simulink model "Mainframe"  (R2021a)
settings: Solver=FixedStepAuto  StartTime=0.0  StopTime=60  FixedStep=0.001  RelTol=1e-3
values from neighbouring files (symbols this model uses):
  den_lpf_d = den_lpf20    [Mainframe_init.m]    (also in load_autopilot.m)
  Emulated_FCC_IO_Delay = 7    [Mainframe_init.m]
  Enable_Gyros = 0    [Mainframe_init.m]
  Enable_INS = 0    [Mainframe_init.m]
  num_lpf_d = num_lpf20    [Mainframe_init.m]    (also in load_autopilot.m)
undefined symbols (not defined in the file or in its folder): act_dmp, act_omega, Actuator, Aerodynamics, aMode, Autopilot, AUX, c_b_WGS, c_be, c_flat, c_grav, c_h_geop0, c_h_geope, c_pa0, c_pe, c_r0, c_rot, c_rsma, c_Tmp0, d_siB_0, d_siB_max, d_siB_min, dd_siB_max, dd_siB_min, dev, DiscIntNeverNeededParam, e_pa, e_Tmp, fin_maxrate, flag_I_act_switch, flag_I_aero_switch, flag_I_flat, flag_I_gravity_switch, flag_I_rot, hcr, HIL_Data, JMMM_0, JMMM_e, JSPB_e, lat_0, lon_0, Mass_Props, mB_0, mM_0, mM_e, National_Instruments, Newton, pBII_0, PCIe, pMPB, pNPB, propellant_kg, prp_FBPB, prp_mdot, prp_T, pSPB, pwm_output1, qEG_0, qIB_0, qIE_0 ... (+31)
libraries: simulink_extras x38, simulink x31, custom_blocks x11, sldrtlib x10, aerolibcommonsys x4, px4Sensorslib x3, px4lib x3, aerolibnav x1
(part 4 of 17)

== system Mainframe/Flight Simulator On/Flat Earth to LLA/LatLong wrap/Latitude Wrap 90 ==
  Lat : Inport
  Abs1 : Abs
  Bias : Bias  Bias=-90
  Bias1 : Bias  Bias=+90
  Compare To Constant : Subsystem  mask(Compare To Constant){relop=>, const=90, OutDataTypeStr=boolean, ZeroCross=on}
      mask prompts: relop "Simulink:masks:Operator_MP"; const "Simulink:masks:ConstantValue_MP"; OutDataTypeStr "Simulink:masks:OutputDataType_MP"; ZeroCross "Simulink:masks:EnableZerocrossingDetection_MP"
      mask help: Simulink:masks:CompareToConstant_MD
      mask init: same as Mainframe/Non-linear Flight Dynamic Model/Stop-Condition/Compare To Constant
      mask TypeOptions relop: == | ~= | < | <= | >= | >
      mask TypeOptions OutDataTypeStr: Simulink:masks:uint8 | Simulink:masks:boolean
      mask Callback ZeroCross: sl('zeroCrossEnable', gcbh);
      mask Display: disp(str)
  Divide1 : Product  Inputs=**
  Gain : Gain  Gain=-1
  Sign1 : Signum
  Switch : Switch  Criteria=u2 ~= 0
  Wrap Angle 180 : Subsystem
      mask init:
      | aeroicon('aeroblk');
  Lat wrapped : Outport  VectorParamsAs1DForOutWhenUnconnected=off
  Wrap flag : Outport  Port=2  VectorParamsAs1DForOutWhenUnconnected=off
  wires:
  Compare To Constant/1(y) -> Switch/2, Wrap flag/1
  Wrap Angle 180/1(Angle 180) -> Sign1/1, Switch/3, Abs1/1
  Lat/1 -> Wrap Angle 180/1(Angle)
  Abs1/1 -> Compare To Constant/1(u), Bias/1
  Bias/1 -> Gain/1
  Gain/1 -> Bias1/1
  Bias1/1 -> Divide1/2
  Sign1/1 -> Divide1/1
  Divide1/1 -> Switch/1
  Switch/1 -> Lat wrapped/1

== system Mainframe/Flight Simulator On/Flat Earth to LLA/LatLong wrap/Wrap Longitude ==
  Angle : Inport
  Abs : Abs
  Bias : Bias  Bias=180
  Bias1 : Bias  Bias=-180
  Compare To Constant : Subsystem  mask(Compare To Constant){relop=>, const=180, OutDataTypeStr=boolean, ZeroCross=on}
      mask prompts: relop "Simulink:masks:Operator_MP"; const "Simulink:masks:ConstantValue_MP"; OutDataTypeStr "Simulink:masks:OutputDataType_MP"; ZeroCross "Simulink:masks:EnableZerocrossingDetection_MP"
      mask help: Simulink:masks:CompareToConstant_MD
      mask init: same as Mainframe/Non-linear Flight Dynamic Model/Stop-Condition/Compare To Constant
      mask TypeOptions relop: == | ~= | < | <= | >= | >
      mask TypeOptions OutDataTypeStr: Simulink:masks:uint8 | Simulink:masks:boolean
      mask Callback ZeroCross: sl('zeroCrossEnable', gcbh);
      mask Display: disp(str)
  Constant2 : Constant  Value=360
  Math Function1 : Math  Operator=mod  SignedPower=on  SaturateOnIntegerOverflow=on
  Switch : Switch  Criteria=u2 ~= 0  Threshold=180
  Angle 180 : Outport  VectorParamsAs1DForOutWhenUnconnected=off
  wires:
  Compare To Constant/1(y) -> Switch/2
  Angle/1 -> Bias/1, Switch/3, Abs/1
  Abs/1 -> Compare To Constant/1(u)
  Bias/1 -> Math Function1/1
  Constant2/1 -> Math Function1/2
  Math Function1/1 -> Bias1/1
  Bias1/1 -> Switch/1
  Switch/1 -> Angle 180/1

== system Mainframe/Flight Simulator On/Flat Earth to LLA/LatLong wrap1/Latitude Wrap 90 ==
  Lat : Inport
  Abs1 : Abs
  Bias : Bias  Bias=-90
  Bias1 : Bias  Bias=+90
  Compare To Constant : Subsystem  mask(Compare To Constant){relop=>, const=90, OutDataTypeStr=boolean, ZeroCross=on}
      mask prompts: relop "Simulink:masks:Operator_MP"; const "Simulink:masks:ConstantValue_MP"; OutDataTypeStr "Simulink:masks:OutputDataType_MP"; ZeroCross "Simulink:masks:EnableZerocrossingDetection_MP"
      mask help: Simulink:masks:CompareToConstant_MD
      mask init: same as Mainframe/Non-linear Flight Dynamic Model/Stop-Condition/Compare To Constant
      mask TypeOptions relop: == | ~= | < | <= | >= | >
      mask TypeOptions OutDataTypeStr: Simulink:masks:uint8 | Simulink:masks:boolean
      mask Callback ZeroCross: sl('zeroCrossEnable', gcbh);
      mask Display: disp(str)
  Divide1 : Product  Inputs=**
  Gain : Gain  Gain=-1
  Sign1 : Signum
  Switch : Switch  Criteria=u2 ~= 0
  Wrap Angle 180 : Subsystem
      mask init:
      | aeroicon('aeroblk');
  Lat wrapped : Outport  VectorParamsAs1DForOutWhenUnconnected=off
  Wrap flag : Outport  Port=2  VectorParamsAs1DForOutWhenUnconnected=off
  wires:
  Compare To Constant/1(y) -> Switch/2, Wrap flag/1
  Wrap Angle 180/1(Angle 180) -> Sign1/1, Switch/3, Abs1/1
  Lat/1 -> Wrap Angle 180/1(Angle)
  Abs1/1 -> Compare To Constant/1(u), Bias/1
  Bias/1 -> Gain/1
  Gain/1 -> Bias1/1
  Bias1/1 -> Divide1/2
  Sign1/1 -> Divide1/1
  Divide1/1 -> Switch/1
  Switch/1 -> Lat wrapped/1

== system Mainframe/Flight Simulator On/Flat Earth to LLA/LatLong wrap1/Wrap Longitude ==
  Angle : Inport
  Abs : Abs
  Bias : Bias  Bias=180
  Bias1 : Bias  Bias=-180
  Compare To Constant : Subsystem  mask(Compare To Constant){relop=>, const=180, OutDataTypeStr=boolean, ZeroCross=on}
      mask prompts: relop "Simulink:masks:Operator_MP"; const "Simulink:masks:ConstantValue_MP"; OutDataTypeStr "Simulink:masks:OutputDataType_MP"; ZeroCross "Simulink:masks:EnableZerocrossingDetection_MP"
      mask help: Simulink:masks:CompareToConstant_MD
      mask init: same as Mainframe/Non-linear Flight Dynamic Model/Stop-Condition/Compare To Constant
      mask TypeOptions relop: == | ~= | < | <= | >= | >
      mask TypeOptions OutDataTypeStr: Simulink:masks:uint8 | Simulink:masks:boolean
      mask Callback ZeroCross: sl('zeroCrossEnable', gcbh);
      mask Display: disp(str)
  Constant2 : Constant  Value=360
  Math Function1 : Math  Operator=mod  SignedPower=on  SaturateOnIntegerOverflow=on
  Switch : Switch  Criteria=u2 ~= 0  Threshold=180
  Angle 180 : Outport  VectorParamsAs1DForOutWhenUnconnected=off
  wires:
  Compare To Constant/1(y) -> Switch/2
  Angle/1 -> Bias/1, Switch/3, Abs/1
  Abs/1 -> Compare To Constant/1(u)
  Bias/1 -> Math Function1/1
  Constant2/1 -> Math Function1/2
  Math Function1/1 -> Bias1/1
  Bias1/1 -> Switch/1
  Switch/1 -> Angle 180/1

== system Mainframe/Flight Simulator On/Flat Earth to LLA/LongLat_offset/Angle Conversion2 ==
  in : Inport  Unit=deg
  Unit Conversion : UnitConversion
  out : Outport  Unit=rad  VectorParamsAs1DForOutWhenUnconnected=off
  wires:
  Unit Conversion/1 -> out/1
  in/1 -> Unit Conversion/1

== system Mainframe/Flight Simulator On/Flat Earth to LLA/LongLat_offset/Find Radian//Distance ==
  mu : Inport
  Angle Conversion2 : Subsystem
  Constant : Constant
  Constant1 : Constant  Value=R
  Constant2 : Constant
  Constant3 : Constant
  Product1 : Product  Inputs=*/  RndMeth=Zero
  Product2 : Product  RndMeth=Zero
  Product3 : Product  Inputs=**/  RndMeth=Zero
  Product4 : Product  RndMeth=Zero
  Sum1 : Sum  Inputs=|+-
  Trigonometric Function : Trigonometry  Operator=cos
  Trigonometric Function1 : Trigonometry  Operator=atan2
  Trigonometric Function2 : Trigonometry  Operator=atan2
  denom : Subsystem
  e : Subsystem
  e^4 : Subsystem
  sqrt : Sqrt  AlgorithmType=Newton-Raphson  SaturateOnIntegerOverflow=on
  dNorth : Outport  VectorParamsAs1DForOutWhenUnconnected=off
  dEast : Outport  Port=2  VectorParamsAs1DForOutWhenUnconnected=off
  wires:
  Angle Conversion2/1(out) -> Trigonometric Function/1, denom/2(mu)
  Trigonometric Function2/1 -> dEast/1
  Trigonometric Function1/1 -> dNorth/1
  Constant3/1 -> Trigonometric Function2/1
  Constant2/1 -> Trigonometric Function1/1
  Product4/1 -> Trigonometric Function2/2
  mu/1 -> Angle Conversion2/1(in)
  Trigonometric Function/1 -> Product4/2
  Product3/1 -> Trigonometric Function1/2  "Rm"
  Sum1/1 -> Product3/2
  Product1/1 -> Product4/1, Product3/1  "Rn"
  Constant/1 -> Sum1/1
  Product2/1 -> Sum1/2
  Constant1/1 -> Product1/1
  sqrt/1 -> Product1/2
  denom/1(denom) -> sqrt/1, Product3/3
  e^4/1(eps) -> Product2/2, Product2/1, denom/1(eps)
  e/1(e) -> e^4/1(e)

== system Mainframe/Flight Table/Flight Table On/Configure Gimbals/Subsystem ==
  Current Stage : Sum  Inputs=3
  One : Constant  OutDataTypeStr=Inherit: Inherit via back propagation
  Stage : Outport
  wires:
  [stage2complete] -> Current Stage/2
  One/1 -> Current Stage/3
  [stage1complete] -> Current Stage/1
  Current Stage/1 -> Stage/1

== system Mainframe/Flight Table/Flight Table On/Configure Gimbals/Ticks To Degrees ==
  In1 : Inport
  Bus Creator : BusCreator  Inputs=3
  Demux : Demux  Outputs=3
  Shaft2degPitch : Gain  Gain=360/(65536)
  Shaft2degRoll : Gain  Gain=-360/(65536)
  Shaft2degYaw : Gain  Gain=360/(65536)
  Out1 : Outport
  wires:
  Shaft2degYaw/1 -> Bus Creator/1  "yawRaw"
  Shaft2degPitch/1 -> Bus Creator/2  "pitchRaw"
  In1/1 -> Demux/1
  Shaft2degRoll/1 -> Bus Creator/3  "rollRaw"
  Bus Creator/1 -> Out1/1
  Demux/2 -> Shaft2degPitch/1  "pitch"
  Demux/1 -> Shaft2degYaw/1  "yaw"
  Demux/3 -> Shaft2degRoll/1  "roll"

== system Mainframe/Non-linear Flight Dynamic Model/Environment/atm_dynamic/trafo_around_z_axis ==
  vec1 : Inport
  gamma : Inport  Port=2
  1_rot_mat : Subsystem  mask(Rotation um 1, 2 oder 3 Achsen){rot_1=Rotation um z-Achse}
      mask prompts: rot_1 "1. Rotation"
      mask help:
      | Dieser Block liefert die Rotationsmatrix T12 für den Fall zurück, dass sich das Ziel-Koordinatensystem (1) durch Drehungen um 1, 2 oder 3 Achsen gegenüber dem Ausgangskoordinatensystem (2) beschreiben lässt (passive Drehung).
      |
      | Die Anzahl der Rotation sowie die Reihenfolge ist frei einstellbar.
      |
      | Die Rotationswinkel haben die Einheit [rad].
      mask TypeOptions rot_1: Rotation um x-Achse | Rotation um y-Achse | Rotation um z-Achse
  Product : Product  Multiplication=Matrix(*)
  Reshape : Reshape  OutputDimensionality=Column vector (2-D)
  vec2 : Outport  VectorParamsAs1DForOutWhenUnconnected=off
  wires:
  Product/1 -> vec2/1  "vec2"
  gamma/1 -> 1_rot_mat/1(wi1)  "gamma"
  1_rot_mat/1(T12) -> Product/1  "T12"
  vec1/1 -> Reshape/1  "vec1"
  Reshape/1 -> Product/2  "vec1"

== system Mainframe/Non-linear Flight Dynamic Model/Extract States/Assemble_States_Bus1/Rotation Angles to Quaternions ==
  "R1, R2, R3" : Inport  Unit=rad
  1/2 : Gain  Gain=0.5  SaturateOnIntegerOverflow=on  OutDataTypeStr=Inherit: Same as input  ParamDataTypeStr=Inherit: Same as input
  Mux1 : Mux  Inputs=2
  Mux2 : Mux
  q0 : Fcn  Expr=u(4)*u(5)*u(6) + u(1)*u(2)*u(3)
  q1 : Fcn  Expr=u(4)*u(5)*u(3) - u(1)*u(2)*u(6)
  q2 : Fcn  Expr=u(4)*u(2)*u(6) + u(1)*u(5)*u(3)
  q3 : Fcn  Expr=u(1)*u(5)*u(6) - u(4)*u(2)*u(3)
  sincos : Trigonometry  Operator=sincos
  Quat : Outport  Unit=1  InitialOutput=0  VectorParamsAs1DForOutWhenUnconnected=off
  wires:
  q0/1 -> Mux2/1
  Mux2/1 -> Quat/1
  q3/1 -> Mux2/4
  q2/1 -> Mux2/3
  q1/1 -> Mux2/2
  Mux1/1 -> q3/1, q2/1, q1/1, q0/1
  sincos/2 -> Mux1/2
  sincos/1 -> Mux1/1
  1/2/1 -> sincos/1
  "R1, R2, R3"/1 -> 1/2/1

== system Mainframe/Non-linear Flight Dynamic Model/Extract States/Assemble_States_Bus1/Three-axis Inertial Measurement Unit3 ==
  A_b : Inport  Unit=m/s^2
  w : Inport  Port=2  Unit=rad/s
  w_dot : Inport  Port=3  Unit=rad/s^2
  CG : Inport  Port=4  Unit=m
  g : Inport  Port=5  Unit=m/s^2
  Acceleration Conversion : Subsystem
  Disallow CGS : UnitConfiguration  UnitSystemsStr=English,SI,SI (extended)  AllowAllUnitSystems=off
  Three-axis Accelerometer : Subsystem  mask(Three-axis Accelerometer){units=Metric (MKS), acc=imu, gtype=on, dtype_a=on, w_a=w_a, z_a=z_a, a_sf_cc=a_sf_cc, a_bias=a_bias, a_Ts=i_Ts, a_rand=on, a_seeds=i_seeds(1:3), a_pow=i_pow(1:3), a_sat=a_sat}
      mask prompts: units "aeroblks:aeroblknav:blockThreeaxisAccelerometerParamUnits"; acc "aeroblks:aeroblknav:blockThreeaxisAccelerometerParamAccelerometerlocation"; gtype "aeroblks:aeroblknav:blockThreeaxisAccelerometerParamSubtractgravity"; dtype_a "aeroblks:aeroblknav:blockThreeaxisAccelerometerParamSecondorderdynamics"; w_a "aeroblks:aeroblknav:blockThreeaxisAccelerometerParamNaturalfrequencyradsec"; z_a "aeroblks:aeroblknav:blockThreeaxisAccelerometerParamDampingratio"; a_sf_cc "aeroblks:aeroblknav:blockThreeaxisAccelerometerParamScalefactorsandcrosscoupling"; a_bias "aeroblks:aeroblknav:blockThreeaxisAccelerometerParamMeasurementbias"; a_Ts "aeroblks:aeroblknav:blockThreeaxisAccelerometerParamUpdateratesec"; a_rand "aeroblks:aeroblknav:blockThreeaxisAccelerometerParamNoiseon"; a_seeds "aeroblks:aeroblknav:blockThreeaxisAccelerometerParamNoiseseeds"; a_pow "aeroblks:aeroblknav:blockThreeaxisAccelerometerParamNoisepower"; a_sat "aeroblks:aeroblknav:blockThreeaxisAccelerometerParamLowerandupperoutputlimits"
      mask help: aeroblks:aeroblknav:blockThreeaxisAccelerometerDesc
      mask init:
      | par = a_Ts;
      | block = gcb;
      | ports=aeroicon('aeroblkaccel','icon',par);
      | a_satl = a_sat(1:3);
      | a_sath = a_sat(4:6);
      mask Help: eval('asbhelp');
      mask TypeOptions units: aeroblks:aeroblknav:blockThreeaxisAccelerometerParamComboMetricMKS | aeroblks:aeroblknav:blockThreeaxisAccelerometerParamComboEnglish
      mask Callback gtype: aeroicon('aeroblkaccel')
      mask Callback dtype_a: aeroicon('aeroblkaccel')
      mask Callback a_rand: aeroicon('aeroblkaccel')
      mask DialogControl ParameterTabVar0 Prompt: Main
      mask DialogControl units Prompt: Units:
      mask DialogControl acc Prompt: Accelerometer location:
      mask DialogControl gtype Prompt: Subtract gravity:
      mask DialogControl dtype_a Prompt: Second-order dynamics
      mask DialogControl w_a Prompt: Natural frequency (rad/sec):
      mask DialogControl z_a Prompt: Damping ratio:
      mask DialogControl a_sf_cc Prompt: Scale factors and cross-coupling:
      mask DialogControl a_bias Prompt: Measurement bias:
      mask DialogControl a_Ts Prompt: Update rate (sec):
      mask DialogControl ParameterTabVar01 Prompt: Noise
      mask DialogControl a_rand Prompt: Noise on
      mask DialogControl a_seeds Prompt: Noise seeds:
      mask DialogControl a_pow Prompt: Noise power:
      mask DialogControl a_sat Prompt: Lower and upper output limits:
      mask Display:
      | port_label(ports(1).type,ports(1).port,ports(1).txt,'texmode','on');
      | port_label(ports(2).type,ports(2).port,ports(2).txt,'texmode','on');
      | port_label(ports(3).type,ports(3).port,ports(3).txt,'texmode','on');
      | port_label(ports(4).type,ports(4).port,ports(4).txt,'texmode','on');
      | port_label(ports(5).type,ports(5).port,ports(5).txt,'texmode','on');
      | port_label(ports(6).type,ports(6).port,ports(6).txt,'texmode','on');
  Three-axis Gyroscope : Subsystem  mask(Three-axis Gyroscope){dtype_g=on, w_g=w_g, z_g=z_g, g_sf_cc=g_sf_cc, g_bias=g_bias, g_sen=g_sens, g_Ts=i_Ts, g_rand=on, g_seeds=i_seeds(4:6), g_pow=i_pow(4:6), g_sat=g_sat}
      mask prompts: dtype_g "aeroblks:aeroblknav:blockThreeaxisGyroscopeParamSecondorderdynamics"; w_g "aeroblks:aeroblknav:blockThreeaxisGyroscopeParamNaturalfrequencyradsec"; z_g "aeroblks:aeroblknav:blockThreeaxisGyroscopeParamDampingratio"; g_sf_cc "aeroblks:aeroblknav:blockThreeaxisGyroscopeParamScalefactorsandcrosscoupling"; g_bias "aeroblks:aeroblknav:blockThreeaxisGyroscopeParamMeasurementbias"; g_sen "aeroblks:aeroblknav:blockThreeaxisGyroscopeParamGsensitivebias"; g_Ts "aeroblks:aeroblknav:blockThreeaxisGyroscopeParamUpdateratesec"; g_rand "aeroblks:aeroblknav:blockThreeaxisGyroscopeParamNoiseon"; g_seeds "aeroblks:aeroblknav:blockThreeaxisGyroscopeParamNoiseseeds"; g_pow "aeroblks:aeroblknav:blockThreeaxisGyroscopeParamNoisepower"; g_sat "aeroblks:aeroblknav:blockThreeaxisGyroscopeParamLowerandupperoutputlimits"
      mask help: aeroblks:aeroblknav:blockThreeaxisGyroscopeDesc
      mask init:
      | par = g_Ts;
      | block = gcb;
      | g_satl = g_sat(1:3);
      | g_sath = g_sat(4:6);
      | ports=aeroicon('aeroblkgyro','icon',par);
      mask Help: eval('asbhelp');
      mask Callback dtype_g: aeroicon('aeroblkgyro');
      mask Callback g_rand: aeroicon('aeroblkgyro');
      mask DialogControl ParameterTabVar0 Prompt: Main
      mask DialogControl dtype_g Prompt: Second-order dynamics
      mask DialogControl w_g Prompt: Natural frequency (rad/sec):
      mask DialogControl z_g Prompt: Damping ratio:
      mask DialogControl g_sf_cc Prompt: Scale factors and cross-coupling:
      mask DialogControl g_bias Prompt: Measurement bias:
      mask DialogControl g_sen Prompt: G-sensitive bias:
      mask DialogControl g_Ts Prompt: Update rate (sec):
      mask DialogControl ParameterTabVar01 Prompt: Noise
      mask DialogControl g_rand Prompt: Noise on
      mask DialogControl g_seeds Prompt: Noise seeds:
      mask DialogControl g_pow Prompt: Noise power:
      mask DialogControl g_sat Prompt: Lower and upper output limits:
      mask Display:
      | port_label(ports(1).type,ports(1).port,ports(1).txt,'texmode','on');
      | port_label(ports(2).type,ports(2).port,ports(2).txt,'texmode','on');
      | port_label(ports(3).type,ports(3).port,ports(3).txt,'texmode','on');
  A_meas : Outport  Unit=m/s^2  VectorParamsAs1DForOutWhenUnconnected=off
  w_meas : Outport  Port=2  Unit=rad/s  VectorParamsAs1DForOutWhenUnconnected=off
  wires:
  Three-axis Accelerometer/1(Ameas) -> A_meas/1
  Three-axis Gyroscope/1((p q r)_meas) -> w_meas/1
  A_b/1 -> Acceleration Conversion/1(acceleration), Three-axis Accelerometer/1(Ab)
  w/1 -> Three-axis Accelerometer/2(p q r), Three-axis Gyroscope/1(p q r)
  CG/1 -> Three-axis Accelerometer/4(CG)
  w_dot/1 -> Three-axis Accelerometer/3(pdot qdot rdot)
  Acceleration Conversion/1(inherit) -> Three-axis Gyroscope/2(G's)
  g/1 -> Three-axis Accelerometer/5(g)

== system Mainframe/Non-linear Flight Dynamic Model/GRM_Airframe/aerodynamics/aerodynamic_via_lookup ==
  pBPB : Inport
  qdynB : Inport  Port=2
  MaB : Inport  Port=3
  alB : Inport  Port=4
  beB : Inport  Port=5
  hBE : Inport  Port=6
  wBIB_star : Inport  Port=7
  afinB : Inport  Port=8
  flag_I_prp : Inport  Port=9
  Bus Creator : BusCreator  Inputs=2
  Demux1 : Demux  Outputs=3
  Demux3 : Demux  Outputs=3
  Gain{,1..4} (5 alike) : Gain  Gain=180/pi
      settings: AttributesFormatString=%<Gain>
  Saturation1 : Saturate  UpperLimit=Aerodynamics.ulim_alpha_deg  LowerLimit=Aerodynamics.llim_alpha_deg
      settings: AttributesFormatString=|
      | %<UpperLimit>
      | %<LowerLimit>
  Saturation4 : Saturate  UpperLimit=Aerodynamics.ulim_beta_deg  LowerLimit=Aerodynamics.llim_beta_deg
      settings: AttributesFormatString=|
      | %<UpperLimit>
      | %<LowerLimit>
  Terminator : Terminator
  Terminator1 : Terminator
  calc_aero_coefficients : Subsystem
  calc_aero_for_mom : Subsystem
  aero_bus : Outport  VectorParamsAs1DForOutWhenUnconnected=off
  wires:
  MaB/1 -> Terminator1/1
  calc_aero_for_mom/1(FBAB) -> Bus Creator/1
  Bus Creator/1 -> aero_bus/1  "aero_bus"
  pBPB/1 -> calc_aero_for_mom/2(pBPB)
  flag_I_prp/1 -> Terminator/1
  hBE/1 -> calc_aero_for_mom/1(hBE)
  calc_aero_for_mom/2(MBAB) -> Bus Creator/2
  qdynB/1 -> calc_aero_for_mom/3(qdynB)
  alB/1 -> Gain3/1
  beB/1 -> Gain4/1
  wBIB_star/1 -> Demux1/1
  Demux1/1 -> calc_aero_coefficients/4(pBIB_star_rps)  "pBIB_star_rps"
  Demux1/2 -> calc_aero_coefficients/5(qBIB_star_rps)  "qBIB_star_rps"
  Demux1/3 -> calc_aero_coefficients/6(rBIB_star_rps)  "rBIB_star_rps"
  afinB/1 -> Demux3/1
  Demux3/2 -> Gain1/1  "etB"
  Demux3/1 -> Gain/1  "xiB"
  Demux3/3 -> Gain2/1  "zeB"
  Gain/1 -> calc_aero_coefficients/1(dela_deg)
  Gain1/1 -> calc_aero_coefficients/2(dele_deg)
  Gain2/1 -> calc_aero_coefficients/3(delr_deg)
  calc_aero_coefficients/1(Cx) -> calc_aero_for_mom/4(Cx)
  calc_aero_coefficients/2(Cy) -> calc_aero_for_mom/5(Cy)
  calc_aero_coefficients/3(Cz) -> calc_aero_for_mom/6(Cz)
  calc_aero_coefficients/4(Cl) -> calc_aero_for_mom/7(Cl)
  calc_aero_coefficients/5(Cm) -> calc_aero_for_mom/8(Cm)
  calc_aero_coefficients/6(Cn) -> calc_aero_for_mom/9(Cn)
  Saturation1/1 -> calc_aero_coefficients/7(alB_deg)
  Saturation4/1 -> calc_aero_coefficients/8(beB_deg)
  Gain3/1 -> Saturation1/1
  Gain4/1 -> Saturation4/1

== system Mainframe/Non-linear Flight Dynamic Model/GRM_Airframe/aerodynamics/logic_base_drag ==
  env_glbl : Inport
  Bus Selector1 : BusSelector  OutputSignals=T_sim_glbl,T_sim_lnch
  Constant : Constant  Value=prp_T(end)
  MATLAB Function : MATLAB Function  TreatAsAtomicUnit=on
  Subtract : Sum  Inputs=+-
  flag_base_drag : Outport  VectorParamsAs1DForOutWhenUnconnected=off
  wires:
  Subtract/1 -> MATLAB Function/1(u)
  Constant/1 -> MATLAB Function/2(t_prp2)
  MATLAB Function/1(flag_base_drag) -> flag_base_drag/1  "flag_base_drag"
  Bus Selector1/1 -> Subtract/1  "<T_sim_glbl>"
  Bus Selector1/2 -> Subtract/2  "<T_sim_lnch>"
  env_glbl/1 -> Bus Selector1/1

== system Mainframe/Non-linear Flight Dynamic Model/GRM_Airframe/environment/WGS84_Gravitation ==
  lon : Inport  PortDimensions=1
  lat : Inport  Port=2  PortDimensions=1
  h : Inport  Port=3  PortDimensions=1
  Assertion : Assertion  AssertionFailFcn="error('WGS84 Gravitationsmodell: Die Werte des Eingangs \"h\" muessen groesser als 0 sein')"
  Assertion1 : Assertion  AssertionFailFcn="error('WGS84 Gravitationsmodell: Die Werte des Eingangs \"Long\" muessen zwischen -180 und +180 liegen')"
  Assertion2 : Assertion  AssertionFailFcn="error('WGS84 Gravitationsmodell: Die Werte des Eingangs \"Lat\" muessen zwischen -90 und +90 liegen')"
  Compare To Constant : simulink/Logic and Bit Operations/Compare To Constant  relop=>=  const=0  OutDataTypeStr=boolean
      settings: SourceProductName=ISim Simulink Block Set
  Interval Test : simulink/Logic and Bit Operations/Interval Test  IntervalClosedRight=on  uplimit=pi  IntervalClosedLeft=on  lowlimit=-pi  OutDataTypeStr=boolean
      settings: SourceProductName=ISim Simulink Block Set
  Interval Test1 : simulink/Logic and Bit Operations/Interval Test  IntervalClosedRight=on  uplimit=pi/2  IntervalClosedLeft=on  lowlimit=-pi/2  OutDataTypeStr=boolean
      settings: SourceProductName=ISim Simulink Block Set
  WGS84_2_ECEF : Subsystem
  WGS84_Gravity_Implementation : MATLAB Function  TreatAsAtomicUnit=on
  gE : Outport  PortDimensions=3  VectorParamsAs1DForOutWhenUnconnected=off
  wires:
  Interval Test1/1 -> Assertion2/1
  Interval Test/1 -> Assertion1/1
  Compare To Constant/1 -> Assertion/1
  WGS84_2_ECEF/1(pE) -> WGS84_Gravity_Implementation/1(pE)  "pE"
  lat/1 -> WGS84_Gravity_Implementation/2(lat_rad), Interval Test1/1, WGS84_2_ECEF/3(lat)  "lat"
  lon/1 -> WGS84_Gravity_Implementation/3(long_rad), Interval Test/1, WGS84_2_ECEF/2(lon)  "lon"
  h/1 -> WGS84_2_ECEF/1(h), Compare To Constant/1  "h"
  WGS84_Gravity_Implementation/1(gamma_R) -> gE/1  "gE"

== system Mainframe/Non-linear Flight Dynamic Model/GRM_Airframe/environment/atmosphere_static_ISO_2533 ==
  hBE : Inport
  env_glbl : Inport  Port=2
  Bus Creator1 : BusCreator  Inputs=6
  Bus Selector1 : BusSelector  OutputSignals=e_Tmp,e_pa
  Saturation : Saturate  UpperLimit=c_h_geope  LowerLimit=c_h_geop0
      settings: AttributesFormatString=|
      | %<UpperLimit>
      | %<LowerLimit>
  density : Subsystem
  geopot_height : Subsystem  mask{mean_earth_radius=c_r0}
      mask prompts: mean_earth_radius "Mean Earth Radius WGS 84 [m]"
      mask TypeOptions mean_earth_radius: mean_earth_radius/Value
  speed_of_sound : Subsystem
  tmp_and_pressure_ISO_2533 : Subsystem
  atm_stat : Outport  VectorParamsAs1DForOutWhenUnconnected=off
  wires:
  speed_of_sound/1(sos) -> Bus Creator1/3
  env_glbl/1 -> Bus Selector1/1
  Bus Selector1/2 -> tmp_and_pressure_ISO_2533/3(e_pa)  "<e_pa>"
  geopot_height/1(h_geop) -> Saturation/1
  Bus Selector1/1 -> tmp_and_pressure_ISO_2533/2(e_Tmp)  "<e_Tmp>"
  Bus Creator1/1 -> atm_stat/1  "atm_stat_bus"
  tmp_and_pressure_ISO_2533/1(Tmp) -> speed_of_sound/1(Tmp), Bus Creator1/4, density/1(Tmp)
  tmp_and_pressure_ISO_2533/2(pa) -> Bus Creator1/6, density/2(pa)
  density/1(rho) -> Bus Creator1/5
  hBE/1 -> Bus Creator1/1, geopot_height/1(hBE)
  Saturation/1 -> Bus Creator1/2, tmp_and_pressure_ISO_2533/1(h_geop)  "h_geop"

== system Mainframe/Non-linear Flight Dynamic Model/GRM_Airframe/environment/convert_to_local_frame ==
  gE : Inport
  Constant1 : Constant  Value=0
  Dot Product : DotProduct  InputSameDT=on  OutDataTypeStr=Inherit: Inherit via internal rule
  Sqrt : Sqrt  SaturateOnIntegerOverflow=on
  Vector Concatenate : Concatenate  NumInputs=3  Mode=Multidimensional array
  gBG : Outport  VectorParamsAs1DForOutWhenUnconnected=off
  wires:
  gE/1 -> Dot Product/1, Dot Product/2
  Constant1/1 -> Vector Concatenate/2, Vector Concatenate/1
  Sqrt/1 -> Vector Concatenate/3
  Vector Concatenate/1 -> gBG/1  "gBG"
  Dot Product/1 -> Sqrt/1

== system Mainframe/Non-linear Flight Dynamic Model/GRM_Airframe/fin_actuators/Rudder ==
  siB_c : Inport
  tRRR : Inport  Port=2
  Add : Sum  Inputs=+-
  Add1 : Sum  Inputs=+-
  Add2 : Sum  Inputs=+++
  Constant1 : Constant  Value=Actuator.fin1_bias
      settings: AttributesFormatString=%<Value>
  Gain : Gain  Gain=omega^2
  Gain2 : Gain  Gain=2*dmp*omega  Multiplication=Matrix(K*u)
  Gain3 : Gain  Gain=unc_bl
  Gain4 : Gain  Gain=Actuator.fin1_scale
      settings: AttributesFormatString=%<Gain>
  Integrator : Integrator  ExternalReset=either  InitialCondition=d_siB_0
  Integrator1 : Integrator  InitialCondition=siB_0  LimitOutput=on  UpperSaturationLimit=siB_max  LowerSaturationLimit=siB_min  ShowSaturationPort=on
  Limiting_Acceleration : MATLAB Function  TreatAsAtomicUnit=on
  Limiting_Rate : MATLAB Function  TreatAsAtomicUnit=on
  Saturation : Saturate  UpperLimit=siB_max  LowerLimit=siB_min
  Saturation1 : Saturate  UpperLimit=siB_max  LowerLimit=siB_min
  Sign : Signum
  siB : Outport  VectorParamsAs1DForOutWhenUnconnected=off
  d_siB : Outport  Port=2  VectorParamsAs1DForOutWhenUnconnected=off
  dd_siB : Outport  Port=3  VectorParamsAs1DForOutWhenUnconnected=off
  wires:
  Saturation1/1 -> siB/1, [siB]  "siB"
  Integrator1/2 -> Integrator/2  "sat"
  Gain4/1 -> Add2/2
  Gain3/1 -> Add2/3
  Sign/1 -> Gain3/1
  tRRR/1 -> Sign/1  "tRRR"
  Integrator1/1 -> Gain4/1, Add/2  "siB"
  Add1/1 -> Limiting_Acceleration/3(dd_siB)  "dd_siB"
  Gain2/1 -> Add1/2
  Gain/1 -> Add1/1
  Add/1 -> Gain/1
  Limiting_Acceleration/1(dd_siB_l) -> Integrator/1, dd_siB/1  "dd_siB_l"
  Limiting_Rate/1(d_siB_l) -> d_siB/1, [d_siB], Integrator1/1  "d_siB_l"
  Integrator/1 -> Limiting_Rate/2(d_siB), Gain2/1  "d_siB"
  Saturation/1 -> Add/1
  Add2/1 -> Saturation1/1
  Constant1/1 -> Add2/1
  siB_c/1 -> Saturation/1  "siB_c"
  [d_siB] -> Limiting_Acceleration/2(d_siB)
  [siB] -> Limiting_Acceleration/1(siB)
  [siB] -> Limiting_Rate/1(siB)

== system Mainframe/Non-linear Flight Dynamic Model/GRM_Airframe/fin_actuators/Rudder1 ==
  siB_c : Inport
  tRRR : Inport  Port=2
  Add : Sum  Inputs=+-
  Add1 : Sum  Inputs=+-
  Add3 : Sum  Inputs=+++
  Constant1 : Constant  Value=Actuator.fin2_bias
      settings: AttributesFormatString=%<Value>
  Gain : Gain  Gain=omega^2
  Gain2 : Gain  Gain=2*dmp*omega  Multiplication=Matrix(K*u)
  Gain3 : Gain  Gain=unc_bl
  Gain4 : Gain  Gain=Actuator.fin2_scale
      settings: AttributesFormatString=%<Gain>
  Integrator : Integrator  ExternalReset=either  InitialCondition=d_siB_0
  Integrator1 : Integrator  InitialCondition=siB_0  LimitOutput=on  UpperSaturationLimit=siB_max  LowerSaturationLimit=siB_min  ShowSaturationPort=on
  Limiting_Acceleration : MATLAB Function  TreatAsAtomicUnit=on
  Limiting_Rate : MATLAB Function  TreatAsAtomicUnit=on
  Saturation : Saturate  UpperLimit=siB_max  LowerLimit=siB_min
  Saturation1 : Saturate  UpperLimit=siB_max  LowerLimit=siB_min
  Sign : Signum
  siB : Outport  VectorParamsAs1DForOutWhenUnconnected=off
  d_siB : Outport  Port=2  VectorParamsAs1DForOutWhenUnconnected=off
  dd_siB : Outport  Port=3  VectorParamsAs1DForOutWhenUnconnected=off
  wires:
  Saturation1/1 -> siB/1, [siB]  "siB"
  Integrator1/2 -> Integrator/2  "sat"
  Gain3/1 -> Add3/3
  Sign/1 -> Gain3/1
  tRRR/1 -> Sign/1  "tRRR"
  Integrator1/1 -> Add/2, Gain4/1  "siB"
  Add1/1 -> Limiting_Acceleration/3(dd_siB)  "dd_siB"
  Gain2/1 -> Add1/2
  Gain/1 -> Add1/1
  Add/1 -> Gain/1
  Limiting_Acceleration/1(dd_siB_l) -> Integrator/1, dd_siB/1  "dd_siB_l"
  Limiting_Rate/1(d_siB_l) -> d_siB/1, [d_siB], Integrator1/1  "d_siB_l"
  Integrator/1 -> Limiting_Rate/2(d_siB), Gain2/1  "d_siB"
  Saturation/1 -> Add/1
  Add3/1 -> Saturation1/1
  siB_c/1 -> Saturation/1  "siB_c"
  [d_siB] -> Limiting_Acceleration/2(d_siB)
  [siB] -> Limiting_Acceleration/1(siB)
  [siB] -> Limiting_Rate/1(siB)
  Constant1/1 -> Add3/1
  Gain4/1 -> Add3/2

== system Mainframe/Non-linear Flight Dynamic Model/GRM_Airframe/fin_actuators/Rudder2 ==
  siB_c : Inport
  tRRR : Inport  Port=2
  Add : Sum  Inputs=+-
  Add1 : Sum  Inputs=+-
  Add3 : Sum  Inputs=+++
  Constant1 : Constant  Value=Actuator.fin3_bias
      settings: AttributesFormatString=%<Value>
  Gain : Gain  Gain=omega^2
  Gain2 : Gain  Gain=2*dmp*omega  Multiplication=Matrix(K*u)
  Gain3 : Gain  Gain=unc_bl
  Gain4 : Gain  Gain=Actuator.fin3_scale
      settings: AttributesFormatString=%<Gain>
  Integrator : Integrator  ExternalReset=either  InitialCondition=d_siB_0
  Integrator1 : Integrator  InitialCondition=siB_0  LimitOutput=on  UpperSaturationLimit=siB_max  LowerSaturationLimit=siB_min  ShowSaturationPort=on
  Limiting_Acceleration : MATLAB Function  TreatAsAtomicUnit=on
  Limiting_Rate : MATLAB Function  TreatAsAtomicUnit=on
  Saturation : Saturate  UpperLimit=siB_max  LowerLimit=siB_min
  Saturation1 : Saturate  UpperLimit=siB_max  LowerLimit=siB_min
  Sign : Signum
  siB : Outport  VectorParamsAs1DForOutWhenUnconnected=off
  d_siB : Outport  Port=2  VectorParamsAs1DForOutWhenUnconnected=off
  dd_siB : Outport  Port=3  VectorParamsAs1DForOutWhenUnconnected=off
  wires:
  Saturation1/1 -> siB/1, [siB]  "siB"
  Integrator1/2 -> Integrator/2  "sat"
  Gain3/1 -> Add3/3
  Sign/1 -> Gain3/1
  tRRR/1 -> Sign/1  "tRRR"
  Integrator1/1 -> Gain4/1, Add/2  "siB"
  Add1/1 -> Limiting_Acceleration/3(dd_siB)  "dd_siB"
  Gain2/1 -> Add1/2
  Gain/1 -> Add1/1
  Add/1 -> Gain/1
  Limiting_Acceleration/1(dd_siB_l) -> Integrator/1, dd_siB/1  "dd_siB_l"
  Limiting_Rate/1(d_siB_l) -> d_siB/1, [d_siB], Integrator1/1  "d_siB_l"
  Integrator/1 -> Limiting_Rate/2(d_siB), Gain2/1  "d_siB"
  Saturation/1 -> Add/1
  Add3/1 -> Saturation1/1
  siB_c/1 -> Saturation/1  "siB_c"
  [d_siB] -> Limiting_Acceleration/2(d_siB)
  [siB] -> Limiting_Acceleration/1(siB)
  [siB] -> Limiting_Rate/1(siB)
  Constant1/1 -> Add3/1
  Gain4/1 -> Add3/2

== system Mainframe/Non-linear Flight Dynamic Model/GRM_Airframe/fin_actuators/Rudder3 ==
  siB_c : Inport
  tRRR : Inport  Port=2
  Add : Sum  Inputs=+-
  Add1 : Sum  Inputs=+-
  Add3 : Sum  Inputs=+++
  Constant1 : Constant  Value=Actuator.fin4_bias
      settings: AttributesFormatString=%<Value>
  Gain : Gain  Gain=omega^2
  Gain2 : Gain  Gain=2*dmp*omega  Multiplication=Matrix(K*u)
  Gain3 : Gain  Gain=unc_bl
  Gain4 : Gain  Gain=Actuator.fin4_scale
      settings: AttributesFormatString=%<Gain>
  Integrator : Integrator  ExternalReset=either  InitialCondition=d_siB_0
  Integrator1 : Integrator  InitialCondition=siB_0  LimitOutput=on  UpperSaturationLimit=siB_max  LowerSaturationLimit=siB_min  ShowSaturationPort=on
  Limiting_Acceleration : MATLAB Function  TreatAsAtomicUnit=on
  Limiting_Rate : MATLAB Function  TreatAsAtomicUnit=on
  Saturation : Saturate  UpperLimit=siB_max  LowerLimit=siB_min
  Saturation1 : Saturate  UpperLimit=siB_max  LowerLimit=siB_min
  Sign : Signum
  siB : Outport  VectorParamsAs1DForOutWhenUnconnected=off
  d_siB : Outport  Port=2  VectorParamsAs1DForOutWhenUnconnected=off
  dd_siB : Outport  Port=3  VectorParamsAs1DForOutWhenUnconnected=off
  wires:
  Saturation1/1 -> siB/1, [siB]  "siB"
  Integrator1/2 -> Integrator/2  "sat"
  Gain3/1 -> Add3/3
  Sign/1 -> Gain3/1
  tRRR/1 -> Sign/1  "tRRR"
  Integrator1/1 -> Gain4/1, Add/2  "siB"
  Add1/1 -> Limiting_Acceleration/3(dd_siB)  "dd_siB"
  Gain2/1 -> Add1/2
  Gain/1 -> Add1/1
  Add/1 -> Gain/1
  Limiting_Acceleration/1(dd_siB_l) -> Integrator/1, dd_siB/1  "dd_siB_l"
  Limiting_Rate/1(d_siB_l) -> d_siB/1, [d_siB], Integrator1/1  "d_siB_l"
  Integrator/1 -> Limiting_Rate/2(d_siB), Gain2/1  "d_siB"
  Saturation/1 -> Add/1
  Add3/1 -> Saturation1/1
  siB_c/1 -> Saturation/1  "siB_c"
  [d_siB] -> Limiting_Acceleration/2(d_siB)
  [siB] -> Limiting_Acceleration/1(siB)
  [siB] -> Limiting_Rate/1(siB)
  Constant1/1 -> Add3/1
  Gain4/1 -> Add3/2

== system Mainframe/Non-linear Flight Dynamic Model/GRM_Airframe/fin_actuators/control_allocation ==
  siB : Inport
  d_siB : Inport  Port=2
  dd_siB : Inport  Port=3
  Constant8 : Constant  Value=Tr3r4
  Product : Product  Multiplication=Matrix(*)
  Product1 : Product  Multiplication=Matrix(*)
  Product2 : Product  Multiplication=Matrix(*)
  Tr3r4 : Outport  VectorParamsAs1DForOutWhenUnconnected=off
  finB : Outport  Port=2  VectorParamsAs1DForOutWhenUnconnected=off
  d_finB : Outport  Port=3  VectorParamsAs1DForOutWhenUnconnected=off
  dd_finB : Outport  Port=4  VectorParamsAs1DForOutWhenUnconnected=off
  wires:
  Product/1 -> finB/1  "afinB"
  Constant8/1 -> Tr3r4/1, Product2/1, Product1/1, Product/1  "Tr3r4"
  siB/1 -> Product/2
  d_siB/1 -> Product1/2
  Product1/1 -> d_finB/1  "d_afinB"
  dd_siB/1 -> Product2/2
  Product2/1 -> dd_finB/1  "dd_afinB"

== system Mainframe/Non-linear Flight Dynamic Model/GRM_Airframe/gravity/launch_rail ==
  gBG_c : Inport
  hBE : Inport  Port=2
  Constant1 : Constant  Value=flag_I_gravity_switch
  Constant3 : Constant  Value=0
  Subtract : Sum  Inputs=++-
  Switch : Switch  Criteria=u2 > Threshold  Threshold=0.05
  Vector Concatenate : Concatenate  NumInputs=3
  initial_altitude : Subsystem
  gBG : Outport  VectorParamsAs1DForOutWhenUnconnected=off
  wires:
  Constant1/1 -> Subtract/2
  hBE/1 -> Subtract/1
  Subtract/1 -> Switch/2
  Constant3/1 -> Vector Concatenate/1, Vector Concatenate/2, Vector Concatenate/3
  Switch/1 -> gBG/1  "gBG"
  Vector Concatenate/1 -> Switch/3
  gBG_c/1 -> Switch/1
  initial_altitude/1(hBE_0) -> Subtract/3

== system Mainframe/Non-linear Flight Dynamic Model/GRM_Airframe/motion_kinematics/calc_motion_kinematics ==
  lat : Inport
  lon : Inport  Port=2
  qIB : Inport  Port=3
  calc_transformation_matrix : Subsystem
  earth_rotation : Subsystem
  wIEE : Outport  VectorParamsAs1DForOutWhenUnconnected=off
  TIE : Outport  Port=2  VectorParamsAs1DForOutWhenUnconnected=off
  TEB : Outport  Port=3  VectorParamsAs1DForOutWhenUnconnected=off
  TGB : Outport  Port=4  VectorParamsAs1DForOutWhenUnconnected=off
  TEG : Outport  Port=5  VectorParamsAs1DForOutWhenUnconnected=off
  wEGG : Outport  Port=6  VectorParamsAs1DForOutWhenUnconnected=off
  TIB : Outport  Port=7  VectorParamsAs1DForOutWhenUnconnected=off
  wires:
  earth_rotation/1(wIEE) -> wIEE/1
  earth_rotation/2(TIE) -> TIE/1
  earth_rotation/5(TEG) -> TEG/1
  earth_rotation/6(wEGG) -> wEGG/1
  lon/1 -> earth_rotation/2(lon)
  lat/1 -> earth_rotation/1(lat)
  earth_rotation/3(qIE) -> calc_transformation_matrix/1(qIE)
  earth_rotation/4(qEG) -> calc_transformation_matrix/2(qEG)
  qIB/1 -> calc_transformation_matrix/3(qIB)
  calc_transformation_matrix/1(TEB) -> TEB/1
  calc_transformation_matrix/2(TGB) -> TGB/1
  calc_transformation_matrix/3(TIB) -> TIB/1

== system Mainframe/Non-linear Flight Dynamic Model/GRM_Airframe/propulsion/prp_look_up ==
  env_glbl_bus : Inport
  Bus Selector1 : BusSelector  OutputSignals=T_sim_glbl,T_sim_lnch
  Constant : Constant  Value=0
  Constant1 : Constant  Value=0
  Saturation : Saturate  UpperLimit=prp_T(end)  LowerLimit=0
      settings: AttributesFormatString=|
      | %<UpperLimit>
      | %<LowerLimit>
  Subtract : Sum  Inputs=+-
  Switch : Switch  Criteria=u2 > Threshold
  Switch1 : Switch  Criteria=u2 > Threshold
  Vector Concatenate : Concatenate  NumInputs=3
  thrust_lookup : Lookup_n-D  NumberOfTableDimensions=1  BreakpointsForDimension1=prp_T  Table=prp_FBPB  ExtrapMethod=Clip  UseLastTableValue=on  InternalRulePriority=Speed  RndMeth=Simplest  InputSameDT=on
  FBPM : Outport  VectorParamsAs1DForOutWhenUnconnected=off
  wires:
  Bus Selector1/2 -> Subtract/2  "<T_sim_lnch>"
  Switch/1 -> Saturation/1, Switch1/2, Switch1/3
  thrust_lookup/1 -> Switch1/1
  Bus Selector1/1 -> Subtract/1  "<T_sim_glbl>"
  env_glbl_bus/1 -> Bus Selector1/1
  Constant/1 -> Switch/3
  Subtract/1 -> Switch/1, Switch/2
  Saturation/1 -> thrust_lookup/1
  Vector Concatenate/1 -> FBPM/1  "FBPM"
  Constant1/1 -> Vector Concatenate/3, Vector Concatenate/2
  Switch1/1 -> Vector Concatenate/1  "a_FBPM"

== system Mainframe/Non-linear Flight Dynamic Model/GRM_Airframe/propulsion/prp_uncertainty ==
  FBPM : Inport
  wab : Inport  Port=2
  3_rot_mat : Subsystem  mask(Rotation um 1, 2 oder 3 Achsen){rot_1=Rotation um z-Achse, rot_2=Rotation um y-Achse, rot_3=Rotation um x-Achse}
      mask prompts: rot_1 "1. Rotation"; rot_2 "2. Rotation"; rot_3 "3. Rotation"
      mask help:
      | Dieser Block liefert die Rotationsmatrix T12 für den Fall zurück, dass sich das Ziel-Koordinatensystem (1) durch Drehungen um 1, 2 oder 3 Achsen gegenüber dem Ausgangskoordinatensystem (2) beschreiben lässt (passive Drehung).
      |
      | Die Anzahl der Rotation sowie die Reihenfolge ist frei einstellbar.
      |
      | Die Rotationswinkel haben die Einheit [rad].
      mask TypeOptions rot_1: Rotation um x-Achse | Rotation um y-Achse | Rotation um z-Achse
      mask TypeOptions rot_2: Rotation um x-Achse | Rotation um y-Achse | Rotation um z-Achse
      mask TypeOptions rot_3: Rotation um x-Achse | Rotation um y-Achse | Rotation um z-Achse
  Bus Selector : BusSelector  OutputSignals=pBPB
  Product : Product  Multiplication=Matrix(*)
  Product1 : Product
  Subtract : Sum  Inputs=+-
  Thrust_rot_z : Constant  Value=unc_prp_z
  cross_product : Subsystem
      mask help: cross product r3 = r1 x r2
      mask Help:
      | Name:
      | 
      |     cross_product
      | 
      | Description:
      | 
      |     This block implements the cross product r3 = r1 x r2.
      | 
      | Inputs  [size] [data type] [unit]:
      | 
      |     vector 1  [3] [double] [-]
      |     vector 2  [3] [double] [-]
      | 
      | Outputs  [size] [data type] [unit]:
      | 
      |     resulting vector  [3] [double] [-]
      mask Display: disp(' r3 = r1 x r2')
  pNPB : Constant  Value=pNPB
  thrust_rot_x : Constant  Value=unc_prp_x
  thrust_rot_y : Constant  Value=unc_prp_y
  uncert_thrust : Constant  Value=unc_prp_scale
  FBPB : Outport  VectorParamsAs1DForOutWhenUnconnected=off
  MBPB : Outport  Port=2  VectorParamsAs1DForOutWhenUnconnected=off
  wires:
  Thrust_rot_z/1 -> 3_rot_mat/1(wi1)
  thrust_rot_x/1 -> 3_rot_mat/3(wi3)
  Product/1 -> cross_product/2(r2), FBPB/1  "FBPB"
  FBPM/1 -> Product1/1
  3_rot_mat/1(T12) -> Product/1
  thrust_rot_y/1 -> 3_rot_mat/2(wi2)
  cross_product/1(r1_x_r2) -> MBPB/1  "MBPB"
  wab/1 -> Bus Selector/1
  Bus Selector/1 -> Subtract/1  "<pBPB>"
  uncert_thrust/1 -> Product1/2
  Product1/1 -> Product/2
  pNPB/1 -> Subtract/2
  Subtract/1 -> cross_product/1(r1)

== system Mainframe/Non-linear Flight Dynamic Model/GRM_Airframe/rb_eom/calc_bus_flight_dyn_bus_entries ==
  mot_kin : Inport
  eom : Inport  Port=2
  Bus Selector : BusSelector  OutputSignals=pBII,vBII,qIB,wBIB,d_wBIB,d_vBII
  Bus Selector1 : BusSelector  OutputSignals=pBII
  Bus Selector3 : BusSelector  OutputSignals=TGB,TIB,TIE
  Constant : Constant  Value=pBII_0
      settings: AttributesFormatString=%<Value>
  Gain : Gain  Gain=-1
  Math Function : Math  Operator=transpose  SignedPower=on  SaturateOnIntegerOverflow=on
  Product{,1..3} (4 alike) : Product  Multiplication=Matrix(*)
  Subsystem2 : Subsystem
  Sum : Sum  Inputs=+-
  eom D1 : InportShadow  Port=2
  q12_from_T12 : Subsystem
      mask help: Transforms a Direction Cosine Matrix into a Quaternion
      mask Help:
      | Name:
      | 
      |     q12_from_T12
      | 
      | Description:
      | 
      |     This block implements the transformation of a direction cosine matrix DCM
      |      into the corresponding quaternion.
      | 
      | Inputs  [size] [data type] [unit]:
      | 
      |     direction cosine matrix T12  [3x3] [double] [-]
      | 
      | Outputs  [size] [data type] [unit]:
      | 
      |     quaternion q12  [4] [double] [-]
      mask Display:
      | %port_label('input', 1, 'T12')
      | %port_label('output', 1, 'q12')
      | disp('DCM \rightarrow q','texmode','on')
  quaternion_to_euler_angles : Subsystem
      mask help: transforms quaternions to Euler angles (roll, pitch, yaw)
      mask Help:
      | Name:
      | 
      |     quaternion_to_euler_angles
      | 
      | Description:
      | 
      |     This block implements the transformation of a quaternion into the
      |     corresponding Euler angles (zyx-sequence, roll, pitch, yaw).
      | 
      | Inputs  [size] [data type] [unit]:
      | 
      |     quaternion  [4] [double] [-]
      | 
      | Outputs  [size] [data type] [unit]:
      | 
      |     roll angle phi  [1] [double] [rad]
      |     pitch angle theta  [1] [double] [rad]
      |     yaw angle psi  [1] [double] [rad]
      mask Display:
      | %disp (' q --> (Phi,Theta,Psi) [rad]')
      | disp('q \rightarrow eu(\Phi;\Theta;\Psi)','texmode','on')
  quaternion_to_euler_angles1 : Subsystem
      mask help: transforms quaternions to Euler angles (roll, pitch, yaw)
      mask Help:
      | Name:
      | 
      |     quaternion_to_euler_angles
      | 
      | Description:
      | 
      |     This block implements the transformation of a quaternion into the
      |     corresponding Euler angles (zyx-sequence, roll, pitch, yaw).
      | 
      | Inputs  [size] [data type] [unit]:
      | 
      |     quaternion  [4] [double] [-]
      | 
      | Outputs  [size] [data type] [unit]:
      | 
      |     roll angle phi  [1] [double] [rad]
      |     pitch angle theta  [1] [double] [rad]
      |     yaw angle psi  [1] [double] [rad]
      mask Display:
      | %disp (' q --> (Phi,Theta,Psi) [rad]')
      | disp('q \rightarrow eu(\Phi;\Theta;\Psi)','texmode','on')
  aBIB : Outport  VectorParamsAs1DForOutWhenUnconnected=off
  lon : Outport  Port=2  VectorParamsAs1DForOutWhenUnconnected=off
  lat : Outport  Port=3  VectorParamsAs1DForOutWhenUnconnected=off
  hBE : Outport  Port=4  VectorParamsAs1DForOutWhenUnconnected=off
  vBII : Outport  Port=5  VectorParamsAs1DForOutWhenUnconnected=off
  qIB : Outport  Port=6  VectorParamsAs1DForOutWhenUnconnected=off
  wBIB : Outport  Port=7  VectorParamsAs1DForOutWhenUnconnected=off
  d_wBIB : Outport  Port=8  VectorParamsAs1DForOutWhenUnconnected=off
  d_vBII : Outport  Port=9  VectorParamsAs1DForOutWhenUnconnected=off
  pBII : Outport  Port=10  VectorParamsAs1DForOutWhenUnconnected=off
  euIB : Outport  Port=11  VectorParamsAs1DForOutWhenUnconnected=off
  vBIB : Outport  Port=12  VectorParamsAs1DForOutWhenUnconnected=off
  qGB : Outport  Port=13  VectorParamsAs1DForOutWhenUnconnected=off
  euGB : Outport  Port=14  VectorParamsAs1DForOutWhenUnconnected=off
  euBG : Outport  Port=15  VectorParamsAs1DForOutWhenUnconnected=off
  pBLG : Outport  Port=16  VectorParamsAs1DForOutWhenUnconnected=off
  wires:
  Bus Selector/1 -> pBII/1, Subsystem2/2(pBII)  "<pBII>"
  mot_kin/1 -> Bus Selector3/1
  Bus Selector3/3 -> Subsystem2/1(TIE)  "<TIE>"
  eom/1 -> Bus Selector/1
  Math Function/1 -> [TBI], Product1/1, Product/1  "TBI"
  Bus Selector3/2 -> Math Function/1  "<TIB>"
  Bus Selector/6 -> Product/2, d_vBII/1  "<d_vBII>"
  Product/1 -> aBIB/1  "aBIB"
  Subsystem2/1(lon) -> lon/1
  Subsystem2/2(lat) -> lat/1
  Subsystem2/3(hBE) -> hBE/1  "hBE"
  Bus Selector/2 -> Product1/2, vBII/1  "<vBII>"
  Bus Selector/3 -> quaternion_to_euler_angles/1(q), qIB/1  "<qIB>"
  Bus Selector/4 -> wBIB/1  "<wBIB>"
  Bus Selector/5 -> d_wBIB/1  "<d_wBIB>"
  quaternion_to_euler_angles/1(eulx) -> euIB/1  "euIB"
  Product1/1 -> vBIB/1  "vBIB"
  Bus Selector3/1 -> [TGB], q12_from_T12/1(T12)  "<TGB>"
  q12_from_T12/1(q12) -> quaternion_to_euler_angles1/1(q), qGB/1  "qGB"
  quaternion_to_euler_angles1/1(eulx) -> euGB/1, Gain/1  "euGB"
  Gain/1 -> euBG/1  "euBG"
  eom D1/1 -> Bus Selector1/1
  Bus Selector1/1 -> Sum/1  "<pBII>"
  Constant/1 -> Sum/2
  Sum/1 -> Product3/2  "pBLI"
  [TGB] -> Product2/1
  [TBI] -> Product2/2
  Product2/1 -> Product3/1  "TGI"
  Product3/1 -> pBLG/1  "pBLG"

== system Mainframe/Non-linear Flight Dynamic Model/GRM_Airframe/rb_eom/eom_6dof ==
  for_mom : Inport
  wab : Inport  Port=2
  Bus Selector1 : BusSelector  OutputSignals=mB,JBBB
  Bus Selector2 : BusSelector  OutputSignals=FBTB,MBTB
  Constant : Constant  Value=[pBII_0; vBII_0; qIB_0; wBIB_0]
  Constant9 : Constant  Value=[0 0 0; 0 0 0; 0 0 0]
  Rigid_Body_EOM_6_DOF : Subsystem  mask{flag_Kraft=FBTB}
      mask prompts: flag_Kraft "Input Kraftvektor"
      mask help:
      | 6DOF-Bewegungsgleichungen im ECI-System mit
      | zeitvariantem Massenträgheitsmoment.
      |
      | Modell Varianten:
      | - Koordinatensystem des Kraftvektor:
      |      FBTI : Inertial System I
      |      FBTB : Körperfestes System B
      mask init:
      | switch flag_Kraft
      |     case 1
      |         port_label_kraft = 'FBTI';
      |     case 2
      |         port_label_kraft = 'FBTB';
      | end
      mask TypeOptions flag_Kraft: FBTI | FBTB
      mask DialogControl Container4 Prompt: Modell Einstellungen
      mask Display:
      | port_label ('input',1,port_label_kraft )
      | port_label ('input',2,'MBTB' )
      | port_label ('input',3,'mB' )
      | port_label ('input',4,'x0' )
      | port_label ('input',5,'JBB' )
      | port_label ('input',6,'d_JBB' )
      | port_label ('output',1,'rb_eom' )
  eom : Outport  VectorParamsAs1DForOutWhenUnconnected=off
  wires:
  Bus Selector2/2 -> Rigid_Body_EOM_6_DOF/2(MBTB)  "<MBTB>"
  Bus Selector2/1 -> Rigid_Body_EOM_6_DOF/1(FBTX)  "<FBTB>"
  Rigid_Body_EOM_6_DOF/1(rb_eom) -> eom/1
  Constant9/1 -> Rigid_Body_EOM_6_DOF/6(d_JBB)
  Bus Selector1/2 -> Rigid_Body_EOM_6_DOF/5(JBB)  "<JBBB>"
  for_mom/1 -> Bus Selector2/1
  Constant/1 -> Rigid_Body_EOM_6_DOF/4(x0)
  Bus Selector1/1 -> Rigid_Body_EOM_6_DOF/3(mB)  "<mB>"
  wab/1 -> Bus Selector1/1

== system Mainframe/Non-linear Flight Dynamic Model/GRM_Airframe/stream_flow/calc_stream_flow ==
  TIB : Inport
  wIEE : Inport  Port=2
  TIE : Inport  Port=3
  VBII : Inport  Port=4
  pBII : Inport  Port=5
  wBIB : Inport  Port=6
  rho : Inport  Port=7
  sos : Inport  Port=8
  hBE : Inport  Port=9
  Bus Creator : BusCreator  Inputs=9
  Math Function : Math  Operator=transpose  SignedPower=on  SaturateOnIntegerOverflow=on
  Product : Product  Multiplication=Matrix(*)
  Subsystem1 : Subsystem
  velocity_vector_transformation : Subsystem
  str_flow : Outport  VectorParamsAs1DForOutWhenUnconnected=off
  wires:
  Subsystem1/4(MaB) -> Bus Creator/4
  Math Function/1 -> Product/1  "TBI"
  Subsystem1/2(be) -> Bus Creator/2  "beB"
  Subsystem1/8(fi) -> Bus Creator/8  "fiB"
  VBII/1 -> velocity_vector_transformation/3(vBII)
  Subsystem1/5(a_vB) -> Bus Creator/5
  Product/1 -> Subsystem1/1(vBEB)  "vBEB"
  Subsystem1/6(wBIB_star) -> Bus Creator/6
  TIE/1 -> velocity_vector_transformation/2(TIE)
  Subsystem1/3(qdynB) -> Bus Creator/3
  velocity_vector_transformation/1(vBEI) -> Product/2
  Subsystem1/7(th) -> Bus Creator/7  "inB"
  Subsystem1/1(al) -> Bus Creator/1  "alB"
  wIEE/1 -> velocity_vector_transformation/1(wIEE)
  Bus Creator/1 -> str_flow/1  "str_flow_bus"
  wBIB/1 -> Subsystem1/2(wBIB)
  hBE/1 -> Bus Creator/9
  sos/1 -> Subsystem1/4(sos)
  rho/1 -> Subsystem1/3(rho)
  TIB/1 -> Math Function/1
  pBII/1 -> velocity_vector_transformation/4(pBII)
